simulink model "lab2b"  (R2014a)
settings: Solver=FixedStepDiscrete  StartTime=0.0  StopTime=Inf  FixedStep=sampletime  RelTol=1e-3
undefined symbols (not defined in the file or in its folder): xx
libraries: dspsrcs4 x3, dspsnks4 x3, dspindex x2, dspvision x1, dspadpt3 x1
settings Model: Creator=micro386  LastModifiedBy=micro386

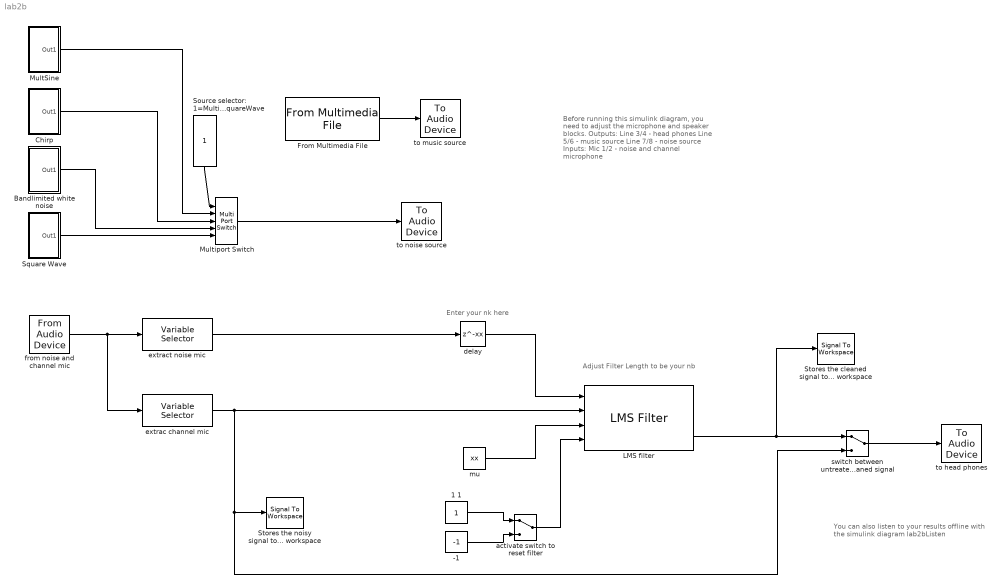
== system lab2b ==
  note: You can also listen to your results offline
      | with the simulink diagram lab2bListen
  note: Enter your nk here
  note: Adjust Filter Length to be your nb
  note: Before running this simulink diagram,
      | you need to adjust the microphone
      | and speaker blocks.
      |
      | Outputs:
      | Line 3/4 - head phones
      | Line 5/6 - music source
      | Line 7/8 - noise source
      |
      | Inputs:
      | Mic 1/2 - noise and channel microphone
  -1 : Constant  Value=-1
  1 1 : Constant
  Bandlimited white noise : Subsystem
  Chirp : Subsystem
  From Multimedia File : dspvision/From Multimedia File  inputFilename=guns.wav  loop=on  numPlays=inf  outputStreams=Audio only  videoDataType=single  audioDataType=double  inheritSampleTime=on  userDefinedSampleTime=1/30  noAudioOutput=off  isIntensityVideo=off  fourcc=RGB  colorVideoFormat=Separate color signals  outputEOF=off  dataOrg=Column-major  audioFrameSize=1024  computeAudioFrameSize=off  outSamplingMode=Frame based
  LMS filter : dspadpt3/LMS Filter  Algo=LMS  L=xx  stepflag=Input port  mu=0.5  leakage=1.0  ic=0  Adapt=off  resetflag=Either edge  weights=off  secondCoeffMode=User-defined  secondCoeffWordLength=2  secondCoeffFracLength=15  accum2Mode=User-defined  accum2FracLength=20  prodOutput2Mode=User-defined  prodOutput2FracLength=20  prodOutput3Mode=User-defined  prodOutput3FracLength=20  prodOutput4Mode=User-defined  prodOutput4FracLength=20  quotientMode=User-defined  quotientFracLength=20  roundingMode=Floor  overflowMode=off  addnparflag=off
  MultSine : Subsystem
  Multiport Switch : MultiPortSwitch  Inputs=4  SaturateOnIntegerOverflow=on  InputSameDT=on
  Source selector: 1=MultiSine 2=Chirp 3=White noise 4=SquareWave : Constant
  Square Wave : Subsystem
  Stores the cleaned signal to the workspace : SignalToWorkspace  VariableName=yCleaned  SaveFormat=Timeseries
      settings: CopyFcn=dspblkcopystw(gcbh);
  Stores the noisy signal to the workspace : SignalToWorkspace  VariableName=yNoisy  SaveFormat=Timeseries
      settings: CopyFcn=dspblkcopystw(gcbh);
  activate switch to reset filter : ManualSwitch
  delay : Delay  DelayLength=xx  InitialCondition=0  InputProcessing=Inherited
  extrac channel mic : dspindex/Variable Selector  NumInputs=1  rowsOrCols=Columns  IdxMode=Fixed  Elements=[2]  ZerOneIdxMode=One-based  errmode=Clip Index  FillMode=on  FillValues=0
  extract noise mic : dspindex/Variable Selector  NumInputs=1  rowsOrCols=Columns  IdxMode=Fixed  Elements=[1]  ZerOneIdxMode=One-based  errmode=Clip Index  FillMode=on  FillValues=0
  from noise and channel mic : dspsrcs4/From Audio Device  deviceName=FCA1616 Mic 1/2 (3- Behringer FCA1616 WDM)  numChannels=2  sampleRate=1/sampletime  deviceDatatype=Determine from output data type  autoBufferSize=on  bufferSize=4096  queueDuration=0.1  frameSize=1  outputDatatype=double  defaultInputChannelMapping=on  inputChannelMapping=1:2
  "mu " : Constant  Value=xx
  switch between untreated and cleaned signal : ManualSwitch
  "to head phones " : dspsnks4/To Audio Device  deviceName=FCA1616 Line 3/4 (3- Behringer FCA1616 WDM)  inheritSampleRate=off  sampleRate=1/sampletime  deviceDatatype=Determine from input data type  autoBufferSize=on  bufferSize=4096  queueDuration=1  defaultOutputChannelMapping=on  outputChannelMapping=1:2
  to music source : dspsnks4/To Audio Device  deviceName=FCA1616 Line 5/6 (3- Behringer FCA1616 WDM)  inheritSampleRate=off  sampleRate=1/sampletime  deviceDatatype=Determine from input data type  autoBufferSize=on  bufferSize=4096  queueDuration=1.0  defaultOutputChannelMapping=on  outputChannelMapping=1:2
  to noise source : dspsnks4/To Audio Device  deviceName=FCA1616 Line 7/8 (3- Behringer FCA1616 WDM)  inheritSampleRate=off  sampleRate=1/sampletime  deviceDatatype=Determine from input data type  autoBufferSize=on  bufferSize=4096  queueDuration=1.0  defaultOutputChannelMapping=on  outputChannelMapping=1:2
  wires:
  Source selector: 1=MultiSine 2=Chirp 3=White noise 4=SquareWave/1 -> Multiport Switch/1
  Chirp/1(Out1) -> Multiport Switch/3
  Square Wave/1(Out1) -> Multiport Switch/5
  Bandlimited white noise/1(Out1) -> Multiport Switch/4
  MultSine/1(Out1) -> Multiport Switch/2
  Multiport Switch/1 -> to noise source/1
  From Multimedia File/1 -> to music source/1
  switch between untreated and cleaned signal/1 -> "to head phones "/1
  "mu "/1 -> LMS filter/3
  delay/1 -> LMS filter/1
  LMS filter/2 -> Stores the cleaned signal to the workspace/1, switch between untreated and cleaned signal/1
  activate switch to reset filter/1 -> LMS filter/4
  1 1/1 -> activate switch to reset filter/1
  -1/1 -> activate switch to reset filter/2
  from noise and channel mic/1 -> extrac channel mic/1, extract noise mic/1
  extract noise mic/1 -> delay/1
  extrac channel mic/1 -> Stores the noisy signal to the workspace/1, switch between untreated and cleaned signal/2, LMS filter/2

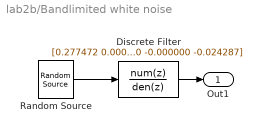
== system lab2b/Bandlimited white noise ==
  Discrete Filter : DiscreteFilter  Numerator=[0.277472 0.000000 -1.387362 0.000000 2.774724 0.000000 -2.774724 0.000000 1.387362 0.000000 -0.277472]*0.3  Denominator=[1.000000 -0.000000 -2.547368 0.000000 2.994845 -0.000000 -1.778046 0.000000 0.534570 -0.000000 -0.024287]  SampleTime=sampletime
  Random Source : dspsrcs4/Random Source  SrcType=Gaussian  NormMethod=Ziggurat  CltLength=12  MinVal=-1  MaxVal=1  MeanVal=0  VarVal=0.6  RepMode=Specify seed  rawSeed=1  IsInherit=off  SampMode=Discrete  SampTime=sampletime  SampFrame=1  DataType=Double  OutComplex=Real
  Out1 : Outport
  wires:
  Discrete Filter/1 -> Out1/1
  Random Source/1 -> Discrete Filter/1

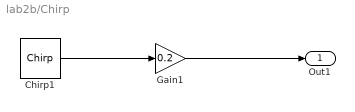
== system lab2b/Chirp ==
  Chirp1 : dspsrcs4/Chirp  sweep=Linear  mode=Bidirectional  f0=600  f1=800  t1=1  Tsweep=10  phase=0  Ts=sampletime  spf=1  datatype=Double
  Gain1 : Gain  Gain=0.2  SaturateOnIntegerOverflow=on  OutDataTypeStr=Inherit: Same as input  ParamDataTypeStr=Inherit: Same as input
  Out1 : Outport
  wires:
  Gain1/1 -> Out1/1
  Chirp1/1 -> Gain1/1

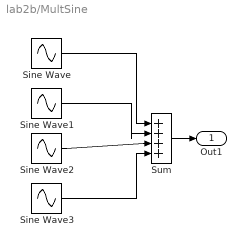
== system lab2b/MultSine ==
  Sine Wave : Sin  Amplitude=.1  Frequency=2*2400  SampleTime=sampletime
  Sine Wave1 : Sin  Amplitude=.1  Frequency=2*3000  SampleTime=sampletime
  Sine Wave2 : Sin  Amplitude=.1  Frequency=2*3600  SampleTime=sampletime
  Sine Wave3 : Sin  Amplitude=.1  Frequency=2*4200  SampleTime=sampletime
  Sum : Sum  Inputs=|++++  SaturateOnIntegerOverflow=on  InputSameDT=on  OutDataTypeStr=Inherit: Same as first input
  Out1 : Outport
  wires:
  Sine Wave/1 -> Sum/1
  Sine Wave1/1 -> Sum/2
  Sine Wave2/1 -> Sum/3
  Sine Wave3/1 -> Sum/4
  Sum/1 -> Out1/1

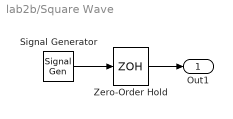
== system lab2b/Square Wave ==
  Signal Generator : SignalGenerator  WaveForm=square  Amplitude=.1  Frequency=100
  Zero-Order Hold : ZeroOrderHold  SampleTime=sampletime
  Out1 : Outport
  wires:
  Zero-Order Hold/1 -> Out1/1
  Signal Generator/1 -> Zero-Order Hold/1
